simulink model "phase_s_R2014a"  (R2014a)
settings: Solver=ode45  SolverMode=SingleTasking  StartTime=0.0  StopTime=20  MaxStep=0.001  RelTol=1e-3
values from neighbouring files (symbols this model uses):
  k = 2    [phase.m]    (also in phase_sin.m)
  T = 1    [phase.m]    (also in phase_sin.m)
  tau = pi/4    (= 0.785398163397)    [phase.m]    (also in phase_sin.m = 3.14159265359)
libraries: simulink x2
settings Model: CovMetricSettings=dwe  CovHtmlReporting=off  covSaveCumulativeToWorkspaceVar=off  CovSaveSingleToWorkspaceVar=off  CovExternalEMLEnable=on  CovSFcnEnable=on  Creator=Witaj Przemku  LastModifiedBy=lev
settings DataIOCC: LimitDataPoints=off  SaveFormat=StructureWithTime
settings DebuggingCC: MergeDetectMultiDrivingBlocksExec=error  SolverPrmCheckMsg=none  FrameProcessingCompatibilityMsg=error  SFUnexpectedBacktrackingDiag=error  SFNoUnconditionalDefaultTransitionDiag=error
settings HardwareCC: ProdBitPerPointer=64  ProdLargestAtomicFloat=Float  ProdIntDivRoundTo=Zero  ProdEndianess=LittleEndian  ProdHWDeviceType=Specified
settings ModelReferenceCC: PropagateSignalLabelsOutOfModel=on
settings GRTTargetCC: TargetLangStandard=C99 (ISO)  GeneratePreprocessorConditionals=Use local settings

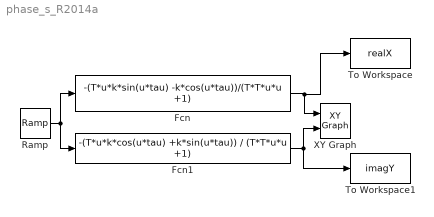
== system phase_s_R2014a ==
  Fcn : Fcn  Expr=-(T*u*k*sin(u*tau) -k*cos(u*tau))/(T*T*u*u +1)
  Fcn1 : Fcn  Expr=-(T*u*k*cos(u*tau) +k*sin(u*tau)) / (T*T*u*u +1)
  Ramp : simulink/Sources/Ramp  slope=1  start=0  X0=0
  To Workspace : ToWorkspace  VariableName=realX  SampleTime=-1
      settings: Save2DSignal=2-D array (concatenate along first dimension)
  To Workspace1 : ToWorkspace  VariableName=imagY  SampleTime=-1
      settings: Save2DSignal=2-D array (concatenate along first dimension)
  XY Graph : simulink/Sinks/XY Graph  xmin=-1  xmax=1  ymin=-1  ymax=1  st=-1
  wires:
  Fcn/1 -> To Workspace/1, XY Graph/1
  Fcn1/1 -> To Workspace1/1, XY Graph/2
  Ramp/1 -> Fcn1/1, Fcn/1
